simulink model "quatercar_model2"  (R2023a)
settings: Solver=VariableStepAuto  StartTime=0.0  StopTime=10.0  RelTol=1e-3
settings Model: Creator=NGOC MAI  LastModifiedBy=NGOC MAI

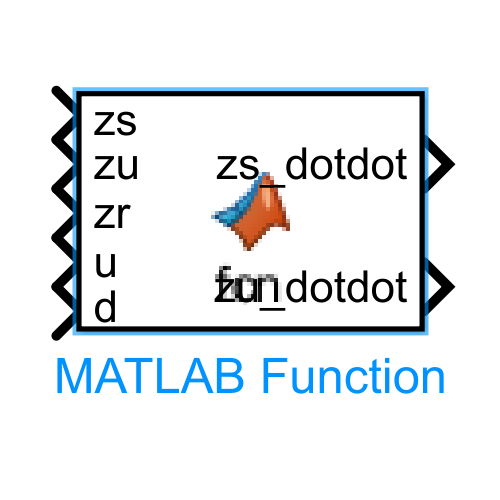
[thumbnail: Simulink's stored preview of the top-level diagram]
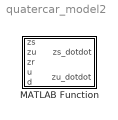
== system quatercar_model2 ==
  MATLAB Function : MATLAB Function  TreatAsAtomicUnit=on

== matlab function quatercar_model2/MATLAB Function ==
  data: zs input; zu input; zr input; u input; zs_dotdot output; d input; zu_dotdot output
function [zs_dotdot,zu_dotdot] = fcn(zs,zu,zr,u,d)
ms=600; %kg
mu=60;%kg
ks=18000; %N/m
ksn=1000; %N/m
bc=2500; Ns/mu
kf=200000; N/m
cf=1000; Ns/m
zs_dotdot=(u+d-fd-fs)/ms;
zu_dotdot=(-u+fd+fs-ft-fb)/mu;

y = u;
